simulink model "ExampleC2"  (Simulink 8.6)
settings: Solver=ode45  StartTime=0.0  StopTime=10.0  RelTol=1e-3
settings Model: Creator=Jacques-Ezechiel  LastModifiedBy=Jacques-Ezechiel
settings DataIOCC: SaveFormat=Dataset  SignalLoggingSaveFormat=Dataset
settings OptimizationCC: ExpressionDepthLimit=128
settings DebuggingCC: UnderspecifiedInitializationDetection=Simplified  MergeDetectMultiDrivingBlocksExec=error  SolverPrmCheckMsg=none  FcnCallInpInsideContextMsg=EnableAllAsError  StateNameClashWarn=none
settings HardwareCC: ProdBitPerPointer=64  ProdLargestAtomicFloat=Float  ProdIntDivRoundTo=Zero  ProdEndianess=LittleEndian  ProdWordSize=64  ProdHWDeviceType=Intel->x86-64 (Windows64)
settings GRTTargetCC: GeneratePreprocessorConditionals=Use local settings  CombineOutputUpdateFcns=on  GRTInterface=off
settings ConfigComp: CovModelRefEnable=off

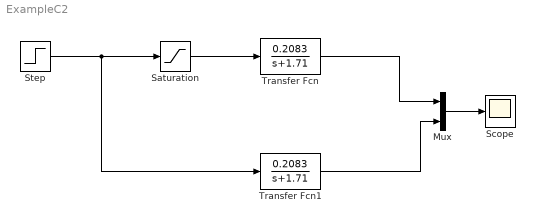
== system ExampleC2 ==
  Mux : Mux  Inputs=2
  Saturation : Saturate  UpperLimit=5  LowerLimit=-5
  Scope : Scope
  Step : Step  Time=0  SampleTime=0
  Transfer Fcn : TransferFcn  Numerator=[0.2083]  Denominator=[1 1.71]
  Transfer Fcn1 : TransferFcn  Numerator=[0.2083]  Denominator=[1 1.71]
  wires:
  Transfer Fcn/1 -> Mux/1
  Transfer Fcn1/1 -> Mux/2
  Saturation/1 -> Transfer Fcn/1
  Step/1 -> Transfer Fcn1/1, Saturation/1
  Mux/1 -> Scope/1
